simulink model "ModelwithSF"  (R2019b)
settings: Solver=VariableStepAuto  StartTime=0.0  StopTime=1500  RelTol=1e-3
values from neighbouring files (symbols this model uses):
  A = [0 -th2 0 th4 0; 0 -1/th3 1/th3 0 0; 0 0 -1/th3 0 0 ... (first row only)    [AugmentedRev1.m]
  A3_c = [0 -th2 th4; 0 -1/th3 0; 0 0 -1/th5]    [AugmentedRev1.m]
  B = [0 0; 0 0; 1/th3 0; 0 0; 0 1/th5]    [AugmentedRev1.m]
  B3_c = [th1 0 0; 0 1/th3 0; 0 0 1/th5]    [AugmentedRev1.m]
  Bc = [th1; 0; 0; 0; 0]    [AugmentedRev1.m]
  C = [1 0 0 0 0]    [AugmentedRev1.m]
  C3_c = [1 0 0; 0 1 0; 0 0 1]    [AugmentedRev1.m]
  D3_c = [0 0 0; 0 0 0; 0 0 0]    [AugmentedRev1.m]
  F3 = [k/th2 -k*th3 (k*th5*th4)/(th2)]    [AugmentedRev1.m]
  Fin = k*[1/th2 -th3 -th3 (th5*th4)/(th2) (th5*th4)/(th2)]    [AugmentedRev1.m]
  th1 = 0.85    [AugmentedRev1.m]
  th2 = 50    [AugmentedRev1.m]
  th3 = 60    [AugmentedRev1.m]
  x0 = [110; th1/th2; th1/th2; 0; 0]    [AugmentedRev1.m]
libraries: dspsrcs4 x1
settings Model: Creator=akshita_jain  LastModifiedBy=akshita_jain

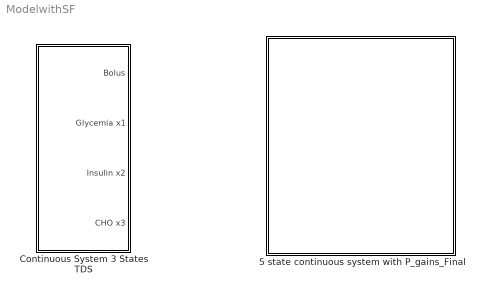
== system ModelwithSF ==
  5 state continuous system with P_gains_Final : Subsystem
  Continuous System 3 States TDS : Subsystem

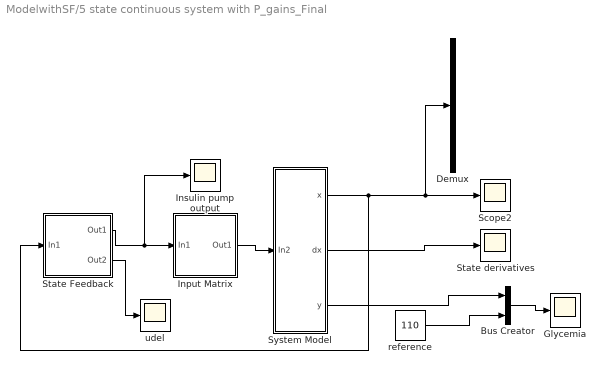
== system ModelwithSF/5 state continuous system with P_gains_Final ==
  Bus Creator : BusCreator  Inputs=2
  Demux : Demux  Outputs=5
  Glycemia : Scope
  Input Matrix : Subsystem
  Insulin pump output : Scope
  Scope2 : Scope
  "State Feedback " : Subsystem
  State derivatives : Scope
  System Model : Subsystem
  reference : Constant  Value=110
  udel : Scope
  wires:
  System Model/3(y) -> Bus Creator/1
  reference/1 -> Bus Creator/2
  System Model/2(dx) -> State derivatives/1
  Bus Creator/1 -> Glycemia/1
  Input Matrix/1(Out1) -> System Model/1(In2)
  "State Feedback "/1(Out1) -> Insulin pump output/1, Input Matrix/1(In1)
  System Model/1(x) -> "State Feedback "/1(In1), Demux/1, Scope2/1
  "State Feedback "/2(Out2) -> udel/1

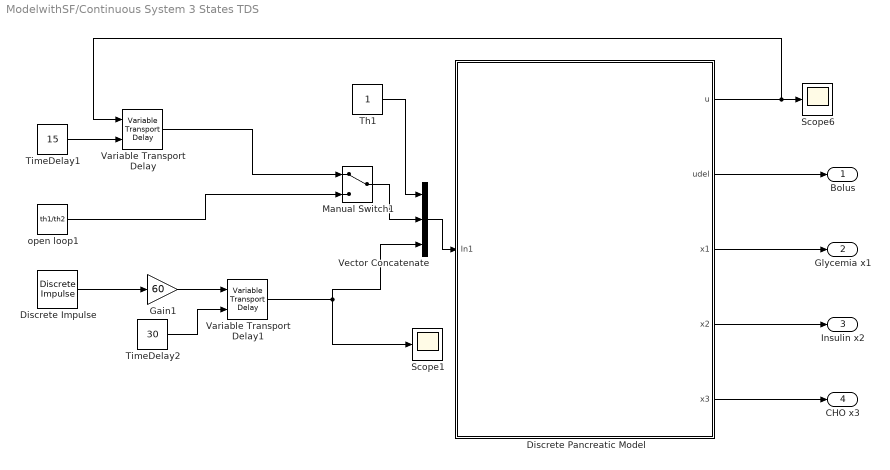
== system ModelwithSF/Continuous System 3 States TDS ==
  Discrete Impulse : dspsrcs4/Discrete  Impulse  Delay=110  SampleTime=1  FrameSample=1  OutputFrames=off  dataType=double  isSigned=on  wordLen=16  udDataType=sfix(16)  fracBitsMode=Best precision  numFracBits=15  OutDataTypeStr=double  LastOutDataTypeStr=double
  Discrete Pancreatic Model : Subsystem
  Gain1 : Gain  Gain=60
  Manual Switch1 : ManualSwitch
  Scope1 : Scope
  Scope6 : Scope
  Th1 : Constant
  TimeDelay1 : Constant  Value=15
  TimeDelay2 : Constant  Value=30
  Variable Transport Delay : VariableTransportDelay  VariableDelayType=Variable transport delay  MaximumDelay=20  InitialOutput=th1/th2
  Variable Transport Delay1 : VariableTransportDelay  VariableDelayType=Variable transport delay  MaximumDelay=40
  Vector Concatenate : Concatenate  NumInputs=3
  open loop1 : Constant  Value=th1/th2
  Bolus : Outport
  Glycemia x1 : Outport  Port=2
  Insulin x2 : Outport  Port=3
  CHO x3 : Outport  Port=4
  wires:
  Discrete Pancreatic Model/3(x1) -> Glycemia x1/1
  Discrete Impulse/1 -> Gain1/1
  Vector Concatenate/1 -> Discrete Pancreatic Model/1(In1)
  Discrete Pancreatic Model/5(x3) -> CHO x3/1
  Discrete Pancreatic Model/4(x2) -> Insulin x2/1
  open loop1/1 -> Manual Switch1/2
  Variable Transport Delay/1 -> Manual Switch1/1
  Variable Transport Delay1/1 -> Vector Concatenate/3, Scope1/1
  Discrete Pancreatic Model/1(u) -> Variable Transport Delay/1, Scope6/1
  Gain1/1 -> Variable Transport Delay1/1
  Th1/1 -> Vector Concatenate/1
  Manual Switch1/1 -> Vector Concatenate/2
  Discrete Pancreatic Model/2(udel) -> Bolus/1
  TimeDelay1/1 -> Variable Transport Delay/2
  TimeDelay2/1 -> Variable Transport Delay1/2

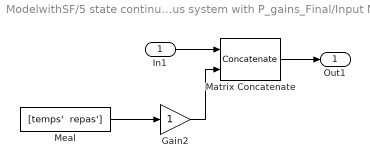
== system ModelwithSF/5 state continuous system with P_gains_Final/Input Matrix ==
  In1 : Inport
  Gain2 : Gain
  Matrix Concatenate : Concatenate  ConcatenateDimension=2
  Meal : FromWorkspace  VariableName="[temps'  repas']"  SampleTime=0
  Out1 : Outport
  wires:
  In1/1 -> Matrix Concatenate/1
  Matrix Concatenate/1 -> Out1/1
  Gain2/1 -> Matrix Concatenate/2
  Meal/1 -> Gain2/1

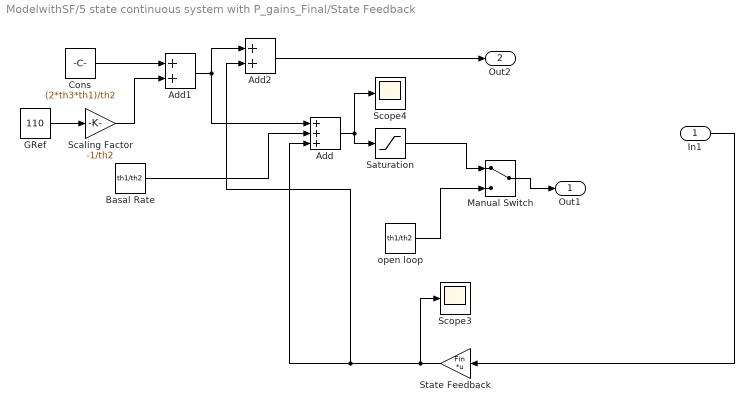
== system ModelwithSF/5 state continuous system with P_gains_Final/State Feedback  ==
  In1 : Inport
  Add : Sum  Inputs=+++
  Add1 : Sum
  Add2 : Sum
  Basal Rate : Constant  Value=th1/th2  VectorParams1D=off
  Cons : Constant  Value=(2*th3*th1)/th2  VectorParams1D=off
  GRef : Constant  Value=110
  Manual Switch : ManualSwitch
  Saturation : Saturate  UpperLimit=2  LowerLimit=0
  Scaling Factor : Gain  Gain=-1/th2
  Scope3 : Scope
  Scope4 : Scope
  State Feedback : Gain  Gain=Fin  Multiplication=Matrix(K*u)
  open loop : Constant  Value=th1/th2
  Out1 : Outport
  Out2 : Outport  Port=2
  wires:
  Manual Switch/1 -> Out1/1
  State Feedback/1 -> Add2/2, Add/3, Scope3/1
  In1/1 -> State Feedback/1
  Scaling Factor/1 -> Add1/2
  Basal Rate/1 -> Add/2
  Add/1 -> Scope4/1, Saturation/1
  open loop/1 -> Manual Switch/2
  GRef/1 -> Scaling Factor/1
  Saturation/1 -> Manual Switch/1
  Add1/1 -> Add/1, Add2/1
  Cons/1 -> Add1/1
  Add2/1 -> Out2/1

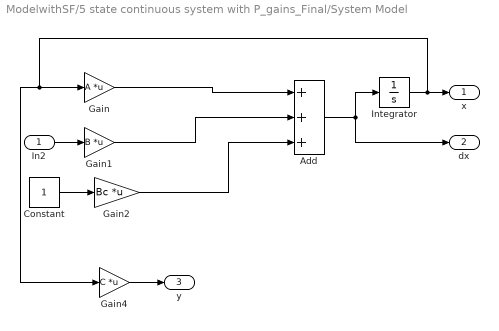
== system ModelwithSF/5 state continuous system with P_gains_Final/System Model ==
  In2 : Inport
  Add : Sum  Inputs=3
  Constant : Constant
  Gain : Gain  Gain=A  Multiplication=Matrix(K*u)
  Gain1 : Gain  Gain=B  Multiplication=Matrix(K*u)
  Gain2 : Gain  Gain=Bc  Multiplication=Matrix(K*u)
  Gain4 : Gain  Gain=C  Multiplication=Matrix(K*u)
  Integrator : Integrator  InitialCondition=x0  ZeroCross=off
  x : Outport
  dx : Outport  Port=2
  y : Outport  Port=3
  wires:
  Gain2/1 -> Add/3
  Gain/1 -> Add/1
  Constant/1 -> Gain2/1
  Integrator/1 -> Gain4/1, Gain/1, x/1
  In2/1 -> Gain1/1
  Add/1 -> Integrator/1, dx/1
  Gain1/1 -> Add/2
  Gain4/1 -> y/1

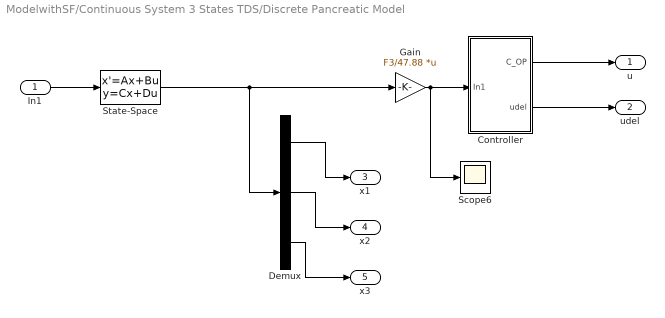
== system ModelwithSF/Continuous System 3 States TDS/Discrete Pancreatic Model ==
  In1 : Inport
  "Controller " : Subsystem
  Demux : Demux  Outputs=3
  Gain : Gain  Gain=F3/47.88  Multiplication=Matrix(K*u)
  Scope6 : Scope
  State-Space : StateSpace  A=A3_c  B=B3_c  C=C3_c  D=D3_c  InitialCondition=[110; th1/th2; 0]
  u : Outport
  udel : Outport  Port=2
  x1 : Outport  Port=3
  x2 : Outport  Port=4
  x3 : Outport  Port=5
  wires:
  "Controller "/1(C_OP) -> u/1
  "Controller "/2(udel) -> udel/1
  State-Space/1 -> Demux/1, Gain/1
  Gain/1 -> Scope6/1, "Controller "/1(In1)
  In1/1 -> State-Space/1
  Demux/1 -> x1/1
  Demux/3 -> x3/1
  Demux/2 -> x2/1

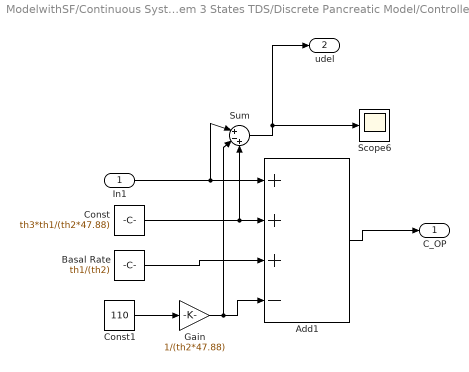
== system ModelwithSF/Continuous System 3 States TDS/Discrete Pancreatic Model/Controller  ==
  In1 : Inport
  Add1 : Sum  Inputs=+++-
  Basal Rate : Constant  Value=th1/(th2)  VectorParams1D=off
  Const : Constant  Value=th3*th1/(th2*47.88)  VectorParams1D=off
  Const1 : Constant  Value=110  VectorParams1D=off
  Gain : Gain  Gain=1/(th2*47.88)
  Scope6 : Scope
  Sum : Sum  Inputs=|+-+
  C_OP : Outport
  udel : Outport  Port=2
  wires:
  Const/1 -> Sum/3, Add1/2
  Basal Rate/1 -> Add1/3
  Add1/1 -> C_OP/1
  Sum/1 -> Scope6/1, udel/1
  In1/1 -> Sum/1, Add1/1
  Const1/1 -> Gain/1
  Gain/1 -> Sum/2, Add1/4
